simulink model "TPPWM_MPCC"  (R2023b)
settings: Solver=VariableStepAuto  StartTime=0.0  StopTime=0.5  RelTol=1e-3
libraries: spsSeriesRLCBranchLib x4, spsVoltageMeasurementLib x4, spsACVoltageSourceLib x3, spsCurrentMeasurementLib x3, slpidlib x1, spsGroundLib x1, spsParallelRLCBranchLib x1, spsUniversalBridgeLib x1, spspowerguiLib x1
settings Model: Creator=17781  LastModifiedBy=ASUS
settings SolverCC: AlgebraicLoopSolver=TrustRegion
settings DataIOCC: ReturnWorkspaceOutputs=off
settings DebuggingCC: UnconnectedInputMsg=warning  UnconnectedOutputMsg=warning  UnconnectedLineMsg=warning
settings ModelReferenceCC: EnableRefExpFcnMdlSchedulingChecks=on
settings SFSimCC: CustomCodeUndefinedFunction=UseInterfaceOnly

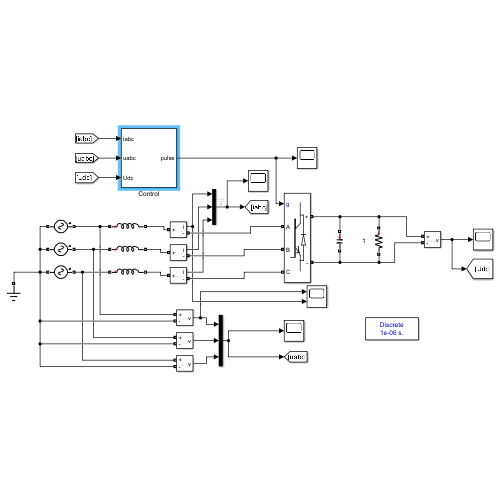
[thumbnail: Simulink's stored preview of the top-level diagram]
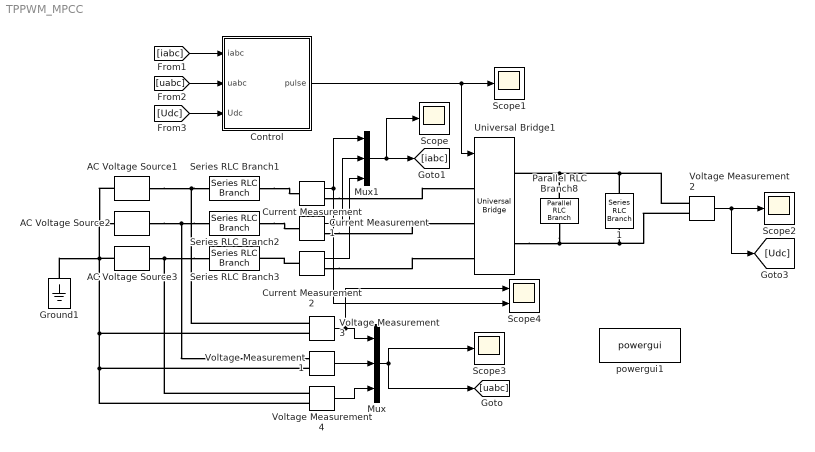
== system TPPWM_MPCC ==
  1 : spsSeriesRLCBranchLib/Series RLC Branch  LConnTagsString=__new0  RConnTagsString=__new0  BranchType=R  Resistance=45  Inductance=0.5e-3  SetiL0=off  InitialCurrent=0  Capacitance=1e-6  Setx0=off  InitialVoltage=0  Measurements=None
  AC Voltage Source1 : spsACVoltageSourceLib/AC Voltage Source  Amplitude=220  Phase=0  Frequency=50  SampleTime=0  Measurements=None  BusType=swing  Pref=10e3  Qref=0  Qmin=-inf  Qmax=+inf
  AC Voltage Source2 : spsACVoltageSourceLib/AC Voltage Source  Amplitude=220  Phase=-120  Frequency=50  SampleTime=0  Measurements=None  BusType=swing  Pref=10e3  Qref=0  Qmin=-inf  Qmax=+inf
  AC Voltage Source3 : spsACVoltageSourceLib/AC Voltage Source  Amplitude=220  Phase=120  Frequency=50  SampleTime=0  Measurements=None  BusType=swing  Pref=10e3  Qref=0  Qmin=-inf  Qmax=+inf
  Control : Subsystem
  Current Measurement : spsCurrentMeasurementLib/Current Measurement  PhasorSimulation=off  OutputType=Complex  PSBequivalent=0
  Current Measurement1 : spsCurrentMeasurementLib/Current Measurement  PhasorSimulation=off  OutputType=Complex  PSBequivalent=0
  Current Measurement2 : spsCurrentMeasurementLib/Current Measurement  PhasorSimulation=off  OutputType=Complex  PSBequivalent=0
  Ground1 : spsGroundLib/Ground  LConnTagsString=a
  Mux : Mux  Inputs=3
  Mux1 : Mux  Inputs=3
  Parallel RLC Branch8 : spsParallelRLCBranchLib/Parallel RLC Branch  LConnTagsString=a  RConnTagsString=__new0  BranchType=C  Resistance=15000  Inductance=1e-3  SetiL0=off  InitialCurrent=0  Capacitance=1100e-6  Setx0=on  InitialVoltage=0  Measurements=None
  Scope{,1..3} (4 alike) : Scope
  Scope4 : Scope  NumInputPorts=2
  Series RLC Branch1 : spsSeriesRLCBranchLib/Series RLC Branch  LConnTagsString=__new0  RConnTagsString=__new0  BranchType=L  Resistance=0.146  Inductance=0.018  SetiL0=off  InitialCurrent=0  Capacitance=1e-6  Setx0=off  InitialVoltage=0  Measurements=None
  Series RLC Branch2 : spsSeriesRLCBranchLib/Series RLC Branch  LConnTagsString=__new0  RConnTagsString=__new0  BranchType=L  Resistance=0.146  Inductance=0.018  SetiL0=off  InitialCurrent=0  Capacitance=1e-6  Setx0=off  InitialVoltage=0  Measurements=None
  Series RLC Branch3 : spsSeriesRLCBranchLib/Series RLC Branch  LConnTagsString=__new0  RConnTagsString=__new0  BranchType=L  Resistance=0.146  Inductance=0.018  SetiL0=off  InitialCurrent=0  Capacitance=1e-6  Setx0=off  InitialVoltage=0  Measurements=None
  Universal Bridge1 : spsUniversalBridgeLib/Universal Bridge  Arms=3  SnubberResistance=1e6  SnubberCapacitance=inf  Device=IGBT / Diodes  Ron=1e-6  Lon=0  ForwardVoltages="[  0  0  ]"  ForwardVoltage=0  GTOparameters=[ 10e-6 , 20e-6 ]  IGBTparameters=[ 1e-6 , 2e-6 ]  Measurements=None  Measurements_2=None  converterType=Rectifier
  Voltage Measurement{1..4} (4 alike) : spsVoltageMeasurementLib/Voltage Measurement  PhasorSimulation=off  OutputType=Complex  PSBequivalent=0
  powergui1 : spspowerguiLib/powergui  Priority=1  SimulationMode=Discrete  SampleTime=1e-6  frequency=60  Iterations=50  frequencyindice=50  Pbase=100e6  ErrMax=1e-4  UnitsV=kV  UnitsW=MW  buscounter=0  FunctionMessages=off  echomessages=off  EnableUseOfTLC=off  CurrentSourceSwitches=off  DisableSnubberDevices=off  DisableRonSwitches=off  DisableVfSwitches=off  DisplayEquations=off  AutomaticDiscreteSolvers=off  SolverType=Tustin/Backward Euler (TBE)  Interpol=off  ExternalGateDelay=off  methode=off  Ts=100  x0status=blocks  SPID=on  SwTol=0  HookPort=off  NonlinearTolerance=0  nMaxIteration=15  ContinueOnMaxIteration=off  RestoreLinks=warning  ResistiveCurrentMeasurement=off  Frange=[0:2:500]  Ylog=off  Xlog=on  ShowGrid=off  save=off  variable=ZData  structure=ScopeData3  ZoomFFT=off  StartTime=0.3  cycles=2  DisplayStyle=1  fundamental=50  FreqAxis=off  MaxFrequency=10000  frequencyindicesteady=1  RmsSteady=1  display=off
  wires:
  Current Measurement2/1 -> Mux1/3
  Voltage Measurement3/1 -> Scope4/1, Mux/1
  Voltage Measurement4/1 -> Mux/3
  [iabc] -> Control/1(iabc)
  Current Measurement/1 -> Mux1/1, Scope4/2
  Control/1(pulse) -> Scope1/1, Universal Bridge1/1
  Mux1/1 -> Scope/1, [iabc]
  Mux/1 -> Scope3/1, [uabc]
  Voltage Measurement1/1 -> Mux/2
  [Udc] -> Control/3(Udc)
  Voltage Measurement2/1 -> Scope2/1, [Udc]
  [uabc] -> Control/2(uabc)
  Current Measurement1/1 -> Mux1/2
  connections:
  1/RConn1 -- Voltage Measurement2/LConn2 -- Universal Bridge1/RConn2 -- Parallel RLC Branch8/RConn1
  Voltage Measurement4/LConn2 -- AC Voltage Source1/LConn1 -- AC Voltage Source2/LConn1 -- Ground1/LConn1 -- AC Voltage Source3/LConn1 -- Voltage Measurement3/LConn2 -- Voltage Measurement1/LConn2
  Series RLC Branch2/RConn1 -- Current Measurement1/LConn1
  Current Measurement2/LConn1 -- Series RLC Branch3/RConn1
  Series RLC Branch3/LConn1 -- AC Voltage Source3/RConn1 -- Voltage Measurement4/LConn1
  Voltage Measurement2/LConn1 -- 1/LConn1 -- Universal Bridge1/RConn1 -- Parallel RLC Branch8/LConn1
  Series RLC Branch1/RConn1 -- Current Measurement/LConn1
  Series RLC Branch2/LConn1 -- AC Voltage Source2/RConn1 -- Voltage Measurement1/LConn1
  Series RLC Branch1/LConn1 -- AC Voltage Source1/RConn1 -- Voltage Measurement3/LConn1
  Current Measurement/RConn1 -- Universal Bridge1/LConn1
  Current Measurement1/RConn1 -- Universal Bridge1/LConn2
  Current Measurement2/RConn1 -- Universal Bridge1/LConn3

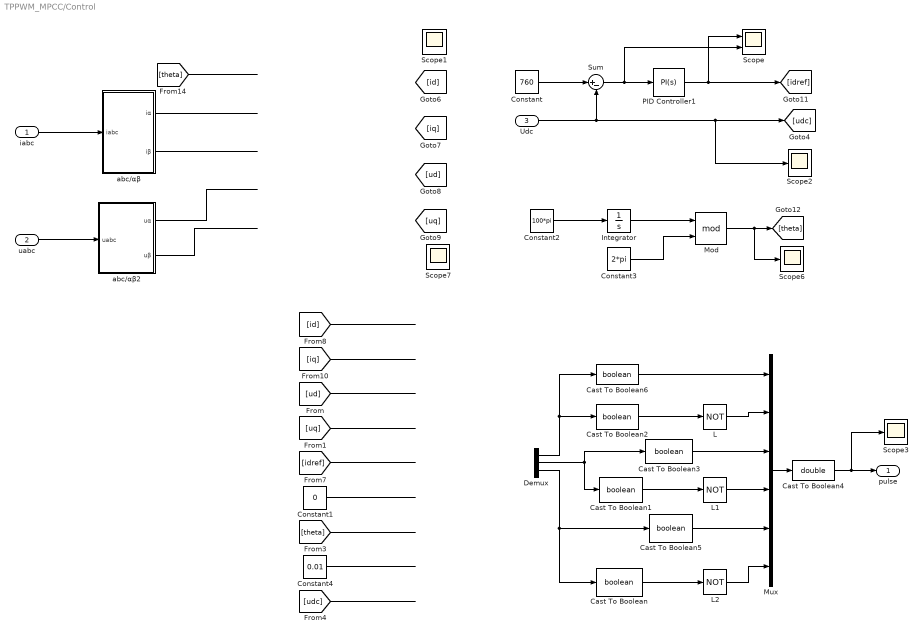
== system TPPWM_MPCC/Control ==
  iabc : Inport
  uabc : Inport  Port=2
  Udc : Inport  Port=3
  Cast To Boolean{,1..3,5..6} (6 alike) : DataTypeConversion  OutDataTypeStr=boolean  SaturateOnIntegerOverflow=off  RndMeth=Floor
  Cast To Boolean4 : DataTypeConversion  OutDataTypeStr=double  SaturateOnIntegerOverflow=off  RndMeth=Floor
  Constant : Constant  Value=760
  Constant1 : Constant  Value=0
  Constant2 : Constant  Value=100*pi
  Constant3 : Constant  Value=2*pi
  Constant4 : Constant  Value=0.01
  Demux : Demux  Outputs=3
  Integrator : Integrator
  L : Logic  Operator=NOT  AllPortsSameDT=off
  L1 : Logic  Operator=NOT  AllPortsSameDT=off
  L2 : Logic  Operator=NOT  AllPortsSameDT=off
  Mod : Math  Operator=mod  SignedPower=on
  Mux : Mux  Inputs=6
  PID Controller1 : slpidlib/PID Controller  Controller=PI  Form=Parallel  TimeDomain=Continuous-time  UseExternalTs=off  SampleTime=-1  IntegratorMethod=Forward Euler  FilterMethod=Forward Euler  ControllerParametersSource=internal  P=0.18  I=4.25  UseKiTs=off  D=0  N=100  UseFilter=on  TunerSelectOption=Transfer Function Based (PID Tuner App)  ZeroCross=off  InitialConditionSource=internal  InitialConditionForIntegrator=0  InitialConditionForFilter=0  DifferentiatorICPrevScaledInput=0  ExternalReset=none  TrackingMode=off  Kt=1  LimitOutput=off  SatLimitsSource=internal  UpperSaturationLimit=inf  LowerSaturationLimit=-inf  LinearizeAsGain=on  AntiWindupMode=none  Kb=1  LimitIntegrator=off  UpperIntegratorSaturationLimit=inf  LowerIntegratorSaturationLimit=-inf  POutMin=[]  POutMax=[]  IOutMin=[]  IOutMax=[]  DOutMin=[]  DOutMax=[]  NOutMin=[]  NOutMax=[]  SumOutMin=[]  SumOutMax=[]  SaturationOutMin=[]  SaturationOutMax=[]  PParamMin=[]  PParamMax=[]  IParamMin=[]  IParamMax=[]  DParamMin=[]  DParamMax=[]  NParamMin=[]  NParamMax=[]  KbParamMin=[]  KbParamMax=[]  KtParamMin=[]  KtParamMax=[]  KbOutMin=[]  KbOutMax=[]  KtOutMin=[]  KtOutMax=[]  IntegratorOutMin=[]  IntegratorOutMax=[]  FilterOutMin=[]  FilterOutMax=[]  SumI1OutMin=[]  SumI1OutMax=[]  SumI2OutMin=[]  SumI2OutMax=[]  SumI3OutMin=[]  SumI3OutMax=[]  SumI4OutMin=[]  SumI4OutMax=[]  SumDOutMin=[]  SumDOutMax=[]  DifferentiatorOutMin=[]  DifferentiatorOutMax=[]  FilterDiffOutCoefMin=[]  FilterDiffOutCoefMax=[]  ReciprocalOutMin=[]  ReciprocalOutMax=[]  SumDenOutMin=[]  SumDenOutMax=[]  SumNumOutMin=[]  SumNumOutMax=[]  DivideOutMin=[]  DivideOutMax=[]  UdiffTsProdOutMin=[]  UdiffTsProdOutMax=[]  NTsProdOutMin=[]  NTsProdOutMax=[]  UintegralTsProdOutMin=[]  UintegralTsProdOutMax=[]  UngainTsProdOutMin=[]  UngainTsProdOutMax=[]  ClampingZeroOutDataTypeStr=Inherit: Inherit via back propagation  ClampingZeroOutMin=[]  ClampingZeroOutMax=[]  FilterDenConstantOutDataTypeStr=Inherit: Inherit via back propagation  FilterDenConstantOutMin=[]  FilterDenConstantOutMax=[]  PCopyOutDataTypeStr=Inherit: Inherit via back propagation  PCopyOutMin=[]  PCopyOutMax=[]  NCopyOutDataTypeStr=Inherit: Inherit via back propagation  NCopyOutMin=[]  NCopyOutMax=[]  IntegratorContinuousStateAttributes=''  IntegratorStateMustResolveToSignalObject=off  IntegratorRTWStateStorageClass=Auto  FilterContinuousStateAttributes=''  FilterStateMustResolveToSignalObject=off  FilterRTWStateStorageClass=Auto  ParallelPVariant=InternalParameters  IdealPVariant=Disabled  IVariant=InternalParameters  DVariant=Disabled  IntegratorVariant=Continuous  SatVariant=Disabled  AWVariant=Passthrough  PCopyVariant=Disabled  TRVariant=Disabled  FdbkBlocksVariant=Forward  IdealPFdbkVariant=Disabled  SatFdbkVariant=Disabled  DerivativeFilterVariant=Disabled  NVariant=Disabled  NCopyVariant=Disabled_SignalSpec  FilterICVariant=Disabled  IntegratorICVariant=InternalICs  ExternalResetVariant=Disabled  TRSumVariant=Passthrough  SumFdbkVariant=Disabled  SumVariant=Sum_PI  TsampFilterVariant=InternalTs  TsampNgainVariant=Passthrough  TsampIntegralVariant=Disabled_SignalSpec  ExternalSaturationOutDataTypeStr=Inherit: Same as second input
  Scope : Scope  NumInputPorts=2
  Scope1 : Scope  NumInputPorts=2
  Scope2 : Scope
  Scope3 : Scope
  Scope6 : Scope
  Scope7 : Scope  NumInputPorts=2
  Sum : Sum  Inputs=|+-
  abc/αβ : Subsystem
  abc/αβ2 : Subsystem
  pulse : Outport  VectorParamsAs1DForOutWhenUnconnected=off
  wires:
  Constant/1 -> Sum/1
  L2/1 -> Mux/6
  Demux/2 -> Cast To Boolean1/1, Cast To Boolean3/1
  L1/1 -> Mux/4
  L/1 -> Mux/2
  Demux/3 -> Cast To Boolean/1, Cast To Boolean5/1
  Constant1/1 -> ?
  Cast To Boolean/1 -> L2/1
  Cast To Boolean1/1 -> L1/1
  Demux/1 -> Cast To Boolean6/1, Cast To Boolean2/1
  Cast To Boolean2/1 -> L/1
  Mux/1 -> Cast To Boolean4/1
  Cast To Boolean3/1 -> Mux/3
  Cast To Boolean5/1 -> Mux/5
  Cast To Boolean6/1 -> Mux/1
  Cast To Boolean4/1 -> Scope3/1, pulse/1
  Sum/1 -> Scope/2, PID Controller1/1
  PID Controller1/1 -> [idref], Scope/1
  Constant2/1 -> Integrator/1
  Integrator/1 -> Mod/1
  Constant3/1 -> Mod/2
  Mod/1 -> Scope6/1, [theta]
  [id] -> ?
  [iq] -> ?
  [ud] -> ?
  [uq] -> ?
  [idref] -> ?
  [theta] -> ?
  Constant4/1 -> ?
  [udc] -> ?
  ? -> Demux/1
  Udc/1 -> Scope2/1, [udc], Sum/2
  iabc/1 -> abc/αβ/1(iabc)
  uabc/1 -> abc/αβ2/1(uabc)
  ? -> Scope1/1, [id]
  ? -> Scope7/2, [uq]
  ? -> Scope1/2, [iq]
  [theta] -> ?
  ? -> Scope7/1, [ud]
  abc/αβ/1(iα) -> ?
  abc/αβ/2(iβ) -> ?
  abc/αβ2/1(uα) -> ?
  abc/αβ2/2(uβ) -> ?

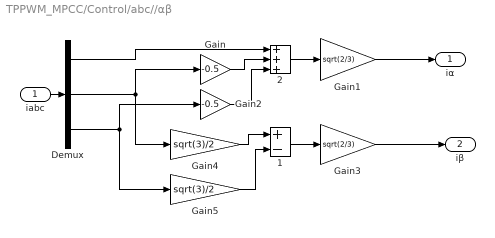
== system TPPWM_MPCC/Control/abc//αβ ==
  iabc : Inport
  "    1" : Sum  Inputs=+-
  "    2" : Sum  Inputs=+++
  Demux : Demux  Outputs=3
  Gain : Gain  Gain=-0.5
  Gain1 : Gain  Gain=sqrt(2/3)
  Gain2 : Gain  Gain=-0.5
  Gain3 : Gain  Gain=sqrt(2/3)
  Gain4 : Gain  Gain=sqrt(3)/2
  Gain5 : Gain  Gain=sqrt(3)/2
  iα : Outport  VectorParamsAs1DForOutWhenUnconnected=off
  iβ : Outport  Port=2  VectorParamsAs1DForOutWhenUnconnected=off
  wires:
  Gain/1 -> "    2"/2
  Gain3/1 -> iβ/1
  Demux/1 -> "    2"/1
  "    2"/1 -> Gain1/1
  iabc/1 -> Demux/1
  Gain1/1 -> iα/1
  Demux/2 -> Gain/1, Gain4/1
  Gain2/1 -> "    2"/3
  Demux/3 -> Gain2/1, Gain5/1
  "    1"/1 -> Gain3/1
  Gain4/1 -> "    1"/1
  Gain5/1 -> "    1"/2

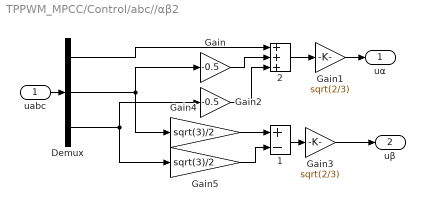
== system TPPWM_MPCC/Control/abc//αβ2 ==
  uabc : Inport
  "    1" : Sum  Inputs=+-
  "    2" : Sum  Inputs=+++
  Demux : Demux  Outputs=3
  Gain : Gain  Gain=-0.5
  Gain1 : Gain  Gain=sqrt(2/3)
  Gain2 : Gain  Gain=-0.5
  Gain3 : Gain  Gain=sqrt(2/3)
  Gain4 : Gain  Gain=sqrt(3)/2
  Gain5 : Gain  Gain=sqrt(3)/2
  uα : Outport  VectorParamsAs1DForOutWhenUnconnected=off
  uβ : Outport  Port=2  VectorParamsAs1DForOutWhenUnconnected=off
  wires:
  Gain5/1 -> "    1"/2
  Gain4/1 -> "    1"/1
  "    1"/1 -> Gain3/1
  Demux/3 -> Gain5/1, Gain2/1
  Gain2/1 -> "    2"/3
  Demux/2 -> Gain4/1, Gain/1
  Gain1/1 -> uα/1
  uabc/1 -> Demux/1
  "    2"/1 -> Gain1/1
  Demux/1 -> "    2"/1
  Gain3/1 -> uβ/1
  Gain/1 -> "    2"/2
